simulink model "Test_mass"  (R2021a)
settings: Solver=VariableStepAuto  StartTime=0.0  StopTime=3600*49  FixedStep=0.01  RelTol=1e-3
libraries: dspsrcs4 x2
settings Model: Creator=verybc  LastModifiedBy=verybc

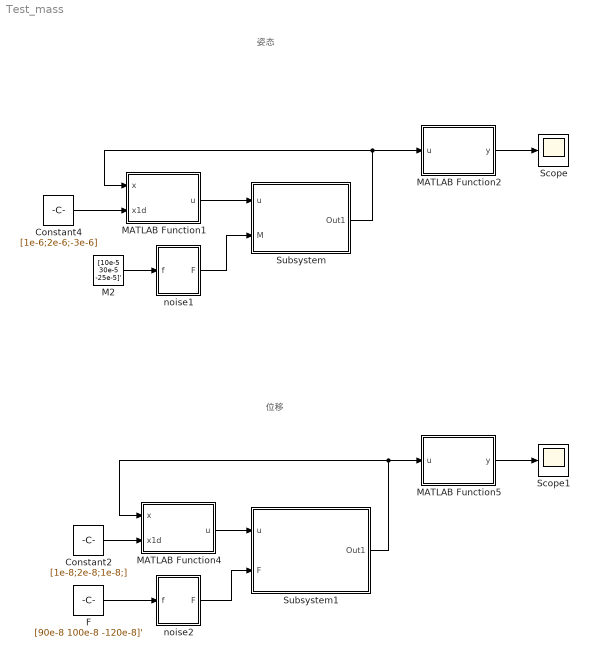
== system Test_mass ==
  note: 位移
  note: 姿态
  Constant2 : Constant  Value=[1e-8;2e-8;1e-8;]
  Constant4 : Constant  Value=[1e-6;2e-6;-3e-6]
  F : Constant  Value=[90e-8 100e-8 -120e-8]'
  M2 : Constant  Value=[10e-5 30e-5 -25e-5]'
  MATLAB Function1 : MATLAB Function  TreatAsAtomicUnit=on
  MATLAB Function2 : MATLAB Function  TreatAsAtomicUnit=on
  MATLAB Function4 : MATLAB Function  TreatAsAtomicUnit=on
  MATLAB Function5 : MATLAB Function  TreatAsAtomicUnit=on
  Scope : Scope
  Scope1 : Scope
  Subsystem : Subsystem
  Subsystem1 : Subsystem
  noise1 : Subsystem
  noise2 : Subsystem
  wires:
  M2/1 -> noise1/1(f)
  MATLAB Function2/1(y) -> Scope/1
  noise1/1(F) -> Subsystem/2(M)
  MATLAB Function1/1(u) -> Subsystem/1(u)
  Subsystem/1(Out1) -> MATLAB Function1/1(x), MATLAB Function2/1(u)
  MATLAB Function5/1(y) -> Scope1/1
  Subsystem1/1(Out1) -> MATLAB Function4/1(x), MATLAB Function5/1(u)
  MATLAB Function4/1(u) -> Subsystem1/1(u)
  F/1 -> noise2/1(f)
  noise2/1(F) -> Subsystem1/2(F)
  Constant4/1 -> MATLAB Function1/2(x1d)
  Constant2/1 -> MATLAB Function4/2(x1d)

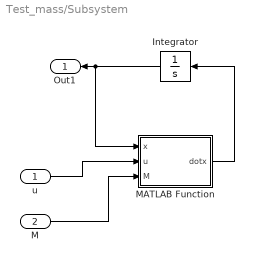
== system Test_mass/Subsystem ==
  u : Inport
  M : Inport  Port=2
  Integrator : Integrator  InitialCondition=[0 0 0 0 0 0]'
  MATLAB Function : MATLAB Function  TreatAsAtomicUnit=on
  Out1 : Outport
  wires:
  MATLAB Function/1(dotx) -> Integrator/1
  u/1 -> MATLAB Function/2(u)
  Integrator/1 -> MATLAB Function/1(x), Out1/1
  M/1 -> MATLAB Function/3(M)

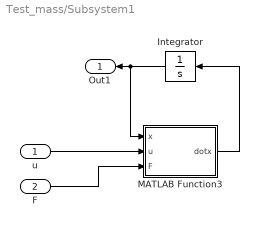
== system Test_mass/Subsystem1 ==
  u : Inport
  F : Inport  Port=2
  Integrator : Integrator  InitialCondition=[0;0;0;0;0;0]
  MATLAB Function3 : MATLAB Function  TreatAsAtomicUnit=on
  Out1 : Outport
  wires:
  MATLAB Function3/1(dotx) -> Integrator/1
  Integrator/1 -> MATLAB Function3/1(x), Out1/1
  u/1 -> MATLAB Function3/2(u)
  F/1 -> MATLAB Function3/3(F)

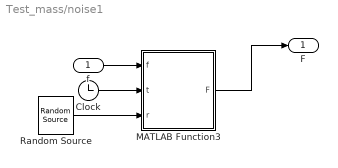
== system Test_mass/noise1 ==
  f : Inport
  Clock : Clock
  MATLAB Function3 : MATLAB Function  TreatAsAtomicUnit=on
  Random Source : dspsrcs4/Random Source  SrcType=Uniform  NormMethod=Ziggurat  CltLength=12  MinVal=0.95  MaxVal=1.05  MeanVal=0  VarVal=1  RepMode=Not repeatable  rawSeed=1  IsInherit=off  SampMode=Discrete  SampTime=1  SampFrame=1  DataType=Double  OutComplex=Real  OutputFrames=off
  F : Outport
  wires:
  f/1 -> MATLAB Function3/1(f)
  MATLAB Function3/1(F) -> F/1
  Clock/1 -> MATLAB Function3/2(t)
  Random Source/1 -> MATLAB Function3/3(r)

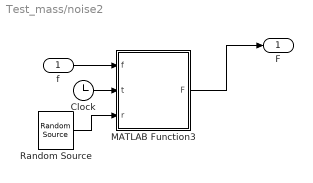
== system Test_mass/noise2 ==
  f : Inport
  Clock : Clock
  MATLAB Function3 : MATLAB Function  TreatAsAtomicUnit=on
  Random Source : dspsrcs4/Random Source  SrcType=Uniform  NormMethod=Ziggurat  CltLength=12  MinVal=0.95  MaxVal=1.05  MeanVal=0  VarVal=1  RepMode=Not repeatable  rawSeed=1  IsInherit=off  SampMode=Discrete  SampTime=1  SampFrame=1  DataType=Double  OutComplex=Real  OutputFrames=off
  F : Outport
  wires:
  Clock/1 -> MATLAB Function3/2(t)
  MATLAB Function3/1(F) -> F/1
  f/1 -> MATLAB Function3/1(f)
  Random Source/1 -> MATLAB Function3/3(r)

== matlab function Test_mass/MATLAB Function1 ==
  data: x input; u output; x1d input
function u = fcn(x,x1d)
s=0.023;
m=1.96;
Ix=m*s^2/12;
Iy=Ix;Iz=Ix;
h=6671000;       %轨道高度
u_=398600e9;     %地心引力常数
w0=(u_/h^3)^0.5; %轨道角速度
A41=-4*w0^2*Ix^-1*(Iy-Iz);
A52=-3*w0^2*Iy^-1*(Ix-Iz);
A63=-w0^2*Iz^-1*(Iy-Ix);
Q=[100 0 0 0 0 0;
    0 100 0 0 0 0;
    0 0 100 0 0 0 ;
    0 0 0 1 0 0;
    0 0 0 0 1 0;
    0 0 0 0 0 1];
R=[1 0 0;
    0 1 0;
    0 0 1;];
K=[-10,0,1.00031740962556e-06,1.00086366037873,0,0;
    0,-10,0,0,1.00086366037871,0;
    -1.00031765377332e-06,0,-10,0,0,1.00086366037871];
e=x1d-x(1:3);
x_=[e;
    x(4:6)];
u = -K*(x_)+[A41*x1d(1,:);
                A52*x1d(2,:);
                A63*x1d(3,:)];

== matlab function Test_mass/Subsystem/MATLAB Function ==
  data: x input; u input; dotx output; M input
function dotx = fcn(x,u,M)
s   = 0.023;                 % 边长
m   = 1.96;                  % 质量
Ix  = m*s^2/12;
Iy  = Ix;
Iz  = Ix;
h   = 6671000;                %轨道高度
u_  = 398600e9;               %地心引力常数
w0  = (u_/h^3)^0.5;           %轨道角速度
A41 = -4*w0^2*Ix^-1*(Iy-Iz);
A46 = -w0*Ix^-1*(Iy-Ix-Iz);
A52 = -3*w0^2*Iy^-1*(Ix-Iz);
A63 = -w0^2*Iz^-1*(Iy-Ix);
A64 = w0*Iz^-1*(Iy-Ix-Iz);
A   = [zeros(3) eye(3);
       A41 0 0 0 0 A46;
       0 A52 0 0 0 0;
       0 0 A63 A64 0 0;];
B   = [zeros(3);
       1/Ix 0 0;
       0 1/Iy 0;
       0 0 1/Iz];
dotx=A*x+B*(u+M);

== matlab function Test_mass/MATLAB Function2 ==
  data: u input; y output
function y = fcn(u)

y = u(1:3);

== matlab function Test_mass/Subsystem1/MATLAB Function3 ==
  data: x input; u input; dotx output; F input
function dotx = fcn(x,u,F)
m    = 1.96;
A    = [zeros(3) eye(3);
        zeros(3,6)];
B    = [zeros(3);
        eye(3)/m];
dotx = A*x+B*(u+F);

== matlab function Test_mass/MATLAB Function4 ==
  data: x input; u output; x1d input
function u = fcn(x,x1d)
m=1.96;

Q=[100 0 0 0 0 0;
    0 100 0 0 0 0;
    0 0 100 0 0 0 ;
    0 0 0 1 0 0;
    0 0 0 0 1 0;
    0 0 0 0 0 1];
R=[1 0 0;
    0 1 0;
    0 0 1;];
K=[-10,0,0,6.34034699365894,0,0;
    0,-10,0,0,6.34034699365894,0;
    0,0,-10,0,0,6.34034699365894];
e=x1d-x(1:3);
x_=[e;
    x(4:6)];
u = -K*(x_);

== matlab function Test_mass/MATLAB Function5 ==
  data: u input; y output
function y = fcn(u)

y = u(1:3);

== matlab function Test_mass/noise2/MATLAB Function3 ==
  data: f input; F output; t input; r input
function F= fcn(f,t,r)

% 低频干扰
F1 = r * (1+0.1 * sin(1/25*t))*f.*[sin(1/2200*t*(sin(1/1510*t)+1.2));
                                   sin(1/2150*t*(sin(1/1500*t)+1.5));
                                   sin(1/2300*t*(sin(1/1525*t)-0.2))];
% 高频干扰
F2 = (r*0.006-0.003)*f.*[sin(1/90*t*(sin(1/51*t)+1.2));
                         sin(1/105*t*(sin(1/70*t)+1.5));
                         sin(1/140*t*(sin(1/25*t)-0.2))];
 
F = F1;

== matlab function Test_mass/noise1/MATLAB Function3 ==
  data: f input; F output; t input; r input
function F= fcn(f,t,r)

F1 =  r * (1+0.1 * sin(1/25*t))* f.*[sin(1/2200 * t * (sin(1/1520*t)+1));
                                     sin(1/2250 * t * (sin(1/1525*t)+1.5));
                                     sin(1/2200 * t * (sin(1/1525*t)+1.2))];

F2 = f.*[sin(1/100*t*(sin(1/50*t)+1));
                         sin(1/125*t*(sin(1/75*t)+0.5));
                         sin(1/150*t*(sin(1/205*t)+0.2))];

F = F1 ;
